simulink model "MX106"  (R2018a)
settings: Solver=VariableStepAuto  StartTime=0.0  StopTime=10.0  RelTol=1e-3
values from neighbouring files (symbols this model uses):
  MX106_amplifier = MX106_supply_voltage/1024    (= 0.014453125)    [MX106_init.m]
  MX106_init_position = 0    [MX106_init.m]
  MX106_Kc = 8e-1    (= 0.8)    [MX106_init.m]
  MX106_Kd = 1/8    (= 0.125)    [MX106_init.m]
  MX106_Ki = 1/1024    (= 0.0009765625)    [MX106_init.m]
  MX106_Kp = 1/4    (= 0.25)    [MX106_init.m]
  MX106_Kv = 9.926e-3    (= 0.009926)    [MX106_init.m]
  MX106_max_speed = 55 * MX106_reduction / 60 * 2 * pi    (= 1468.69456555)    [MX106_init.m]
  MX106_reduction = 255    [MX106_init.m]
  MX106_stall_current = 6.3    [MX106_init.m]
  MX106_stall_torque = 10.0 / MX106_reduction    (= 0.0392156862745)    [MX106_init.m]
  MX106_Te = 1/1000    (= 0.001)    [MX106_init.m]
undefined symbols (not defined in the file or in its folder): MX106_position_gain, MX106_position_offset, MX106_resistor, MX106_speed_gain
libraries: simulink x4, simulink_extras x1, peGeneralControl x1
settings Model: Creator=matt  LastModifiedBy=matt

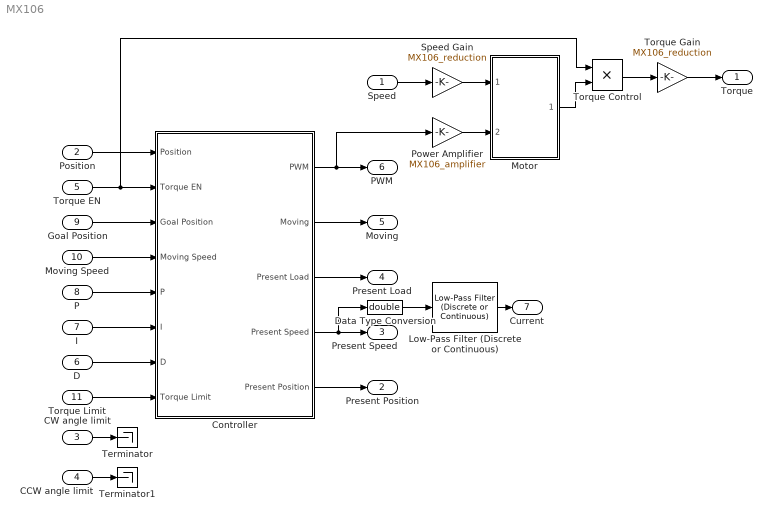
== system MX106 ==
  Speed : Inport
  Position : Inport  Port=2
  CW angle limit : Inport  Port=3  OutDataTypeStr=int16
  CCW angle limit : Inport  Port=4  OutDataTypeStr=int16
  Torque EN : Inport  Port=5  OutDataTypeStr=boolean
  D : Inport  Port=6  OutDataTypeStr=uint8
  I : Inport  Port=7  OutDataTypeStr=uint8
  P : Inport  Port=8  OutDataTypeStr=uint8
  Goal Position : Inport  Port=9
  Moving Speed : Inport  Port=10  OutDataTypeStr=int16
  Torque Limit : Inport  Port=11  OutDataTypeStr=int16
  Controller : Subsystem
  Data Type Conversion : DataTypeConversion  OutDataTypeStr=double
  Low-Pass Filter (Discrete or Continuous) : peGeneralControl/Low-Pass Filter (Discrete or Continuous)  K=9.22996525339537E-07  T=1  B=inf  A=-inf  Ts=-1
  Motor : Subsystem
  Power Amplifier : Gain  Gain=MX106_amplifier  OutDataTypeStr=double
  Speed Gain : Gain  Gain=MX106_reduction
  Terminator : Terminator
  Terminator1 : Terminator
  Torque Control : Product
  Torque Gain : Gain  Gain=MX106_reduction
  Torque : Outport
  Present Position : Outport  Port=2
  Present Speed : Outport  Port=3
  Present Load : Outport  Port=4
  Moving : Outport  Port=5
  PWM : Outport  Port=6
  Current : Outport  Port=7
  wires:
  CW angle limit/1 -> Terminator/1
  CCW angle limit/1 -> Terminator1/1
  Position/1 -> Controller/1(Position)
  Torque EN/1 -> Controller/2(Torque EN), Torque Control/1
  P/1 -> Controller/5(P)
  I/1 -> Controller/6(I)
  D/1 -> Controller/7(D)
  Moving Speed/1 -> Controller/4(Moving Speed)
  Torque Limit/1 -> Controller/8(Torque Limit)
  Controller/2(Moving) -> Moving/1
  Controller/3(Present Load) -> Present Load/1
  Controller/4(Present Speed) -> Data Type Conversion/1, Present Speed/1
  Controller/5(Present Position) -> Present Position/1
  Controller/1(PWM) -> Power Amplifier/1, PWM/1
  Torque Control/1 -> Torque Gain/1
  Speed/1 -> Speed Gain/1
  Speed Gain/1 -> Motor/1(Speed)
  Power Amplifier/1 -> Motor/2(Voltage)
  Motor/1(Torque) -> Torque Control/2
  Goal Position/1 -> Controller/3(Goal Position)
  Torque Gain/1 -> Torque/1
  Low-Pass Filter (Discrete or Continuous)/1 -> Current/1
  Data Type Conversion/1 -> Low-Pass Filter (Discrete or Continuous)/1

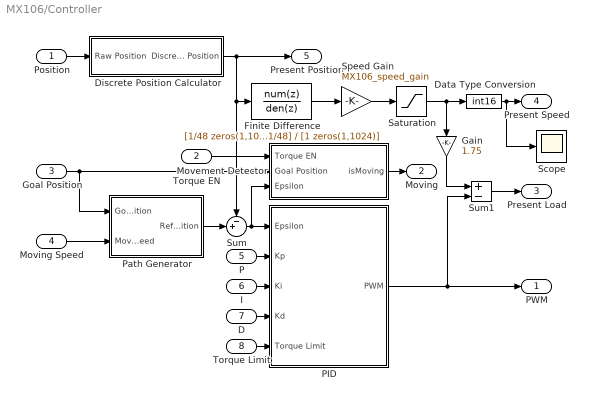
== system MX106/Controller ==
  Position : Inport
  Torque EN : Inport  Port=2
  Goal Position : Inport  Port=3  OutDataTypeStr=int16
  Moving Speed : Inport  Port=4
  P : Inport  Port=5
  I : Inport  Port=6
  D : Inport  Port=7
  Torque Limit : Inport  Port=8
  Data Type Conversion : DataTypeConversion  OutDataTypeStr=int16
  Discrete Position Calculator : Subsystem
  Finite Difference : DiscreteTransferFcn  Numerator=[1/48 zeros(1,1023) -1/48]  Denominator=[1 zeros(1,1024)]  InitialStates=(MX106_init_position + MX106_position_offset) * MX106_position_gain  a0EqualsOne=on
  Gain : Gain  Gain=1.75  OutDataTypeStr=int16
  Movement Detector : Subsystem
  PID : Subsystem
  Path Generator : Subsystem
  Saturation : Saturate  UpperLimit=1024  LowerLimit=-1024  ZeroCross=off
  Scope : Scope
  Speed Gain : Gain  Gain=MX106_speed_gain  OutDataTypeStr=double
  Sum : Sum  Inputs=-+|  AccumDataTypeStr=double  OutMin=-4095  OutMax=4095  OutDataTypeStr=int16  SaturateOnIntegerOverflow=on
  Sum1 : Sum  Inputs=+-
  PWM : Outport
  Moving : Outport  Port=2
  Present Load : Outport  Port=3
  Present Speed : Outport  Port=4
  Present Position : Outport  Port=5
  wires:
  Finite Difference/1 -> Speed Gain/1
  Movement Detector/1(isMoving) -> Moving/1
  Torque EN/1 -> Movement Detector/1(Torque EN)
  Path Generator/1(Ref Position) -> Sum/2
  Moving Speed/1 -> Path Generator/2(Moving Speed)
  Sum/1 -> Movement Detector/3(Epsilon), PID/1(Epsilon)
  Gain/1 -> Sum1/1
  Sum1/1 -> Present Load/1
  P/1 -> PID/2(Kp)
  I/1 -> PID/3(Ki)
  D/1 -> PID/4(Kd)
  Torque Limit/1 -> PID/5(Torque Limit)
  PID/1(PWM) -> Sum1/2, PWM/1
  Data Type Conversion/1 -> Scope/1, Present Speed/1
  Goal Position/1 -> Path Generator/1(Goal Position), Movement Detector/2(Goal Position)
  Discrete Position Calculator/1(Discrete Position) -> Sum/1, Finite Difference/1, Present Position/1
  Position/1 -> Discrete Position Calculator/1(Raw Position)
  Speed Gain/1 -> Saturation/1
  Saturation/1 -> Gain/1, Data Type Conversion/1

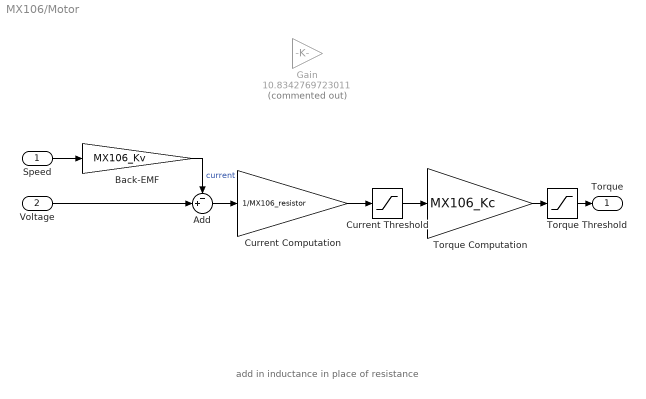
== system MX106/Motor ==
  note: add in inductance in place of resistance
  Speed : Inport
  Voltage : Inport  Port=2
  Add : Sum  Inputs=-+|
  Back-EMF : Gain  Gain=MX106_Kv
  Current Computation : Gain  Gain=1/MX106_resistor
  Current Threshold : Saturate  UpperLimit=MX106_stall_current  LowerLimit=-MX106_stall_current  ZeroCross=off
  Gain : Gain  Commented=on  Gain=10.8342769723011
  Torque Computation : Gain  Gain=MX106_Kc
  Torque Threshold : Saturate  UpperLimit=MX106_stall_torque  LowerLimit=-MX106_stall_torque  ZeroCross=off
  Torque : Outport
  wires:
  Voltage/1 -> Add/2
  Add/1 -> Current Computation/1
  Torque Threshold/1 -> Torque/1
  Current Computation/1 -> Current Threshold/1
  Torque Computation/1 -> Torque Threshold/1
  Current Threshold/1 -> Torque Computation/1
  Back-EMF/1 -> Add/1  "current"
  Speed/1 -> Back-EMF/1

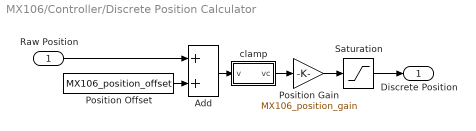
== system MX106/Controller/Discrete Position Calculator ==
  Raw Position : Inport
  Add : Sum
  Position Gain : Gain  Gain=MX106_position_gain  OutMin=0  OutMax=4096  OutDataTypeStr=int16  SampleTime=MX106_Te  SaturateOnIntegerOverflow=on
  Position Offset : Constant  Value=MX106_position_offset
  Saturation : Saturate  UpperLimit=4095  LowerLimit=0  ZeroCross=off
  clamp : Subsystem
  Discrete Position : Outport
  wires:
  Position Gain/1 -> Saturation/1
  Position Offset/1 -> Add/2
  Raw Position/1 -> Add/1
  Saturation/1 -> Discrete Position/1
  Add/1 -> clamp/1(v)
  clamp/1(vc) -> Position Gain/1

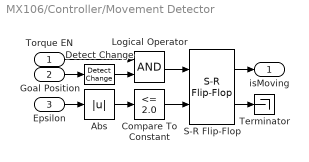
== system MX106/Controller/Movement Detector ==
  Torque EN : Inport
  Goal Position : Inport  Port=2
  Epsilon : Inport  Port=3
  Abs : Abs  ZeroCross=off
  Compare To Constant : simulink/Logic and Bit Operations/Compare To Constant  relop=<=  const=2.0  OutDataTypeStr=boolean  ZeroCross=off
  Detect Change : simulink/Logic and Bit Operations/Detect Change  vinit=0  OutDataTypeStr=boolean
  Logical Operator : Logic  AllPortsSameDT=off  OutDataTypeStr=boolean
  S-R Flip-Flop : simulink_extras/Flip Flops/S-R Flip-Flop  initial_condition=0
  Terminator : Terminator
  isMoving : Outport
  wires:
  Compare To Constant/1 -> S-R Flip-Flop/2
  Abs/1 -> Compare To Constant/1
  Goal Position/1 -> Detect Change/1
  Detect Change/1 -> Logical Operator/2
  S-R Flip-Flop/2 -> Terminator/1
  Logical Operator/1 -> S-R Flip-Flop/1
  Epsilon/1 -> Abs/1
  S-R Flip-Flop/1 -> isMoving/1
  Torque EN/1 -> Logical Operator/1

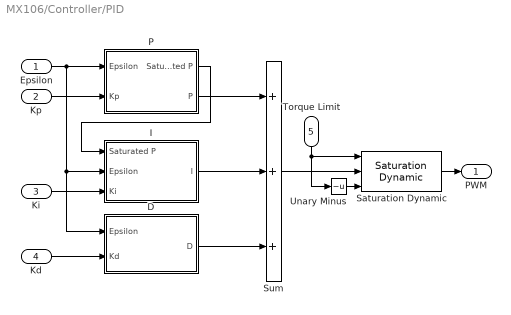
== system MX106/Controller/PID ==
  Epsilon : Inport
  Kp : Inport  Port=2
  Ki : Inport  Port=3
  Kd : Inport  Port=4
  Torque Limit : Inport  Port=5
  D : Subsystem
  I : Subsystem
  P : Subsystem
  Saturation Dynamic : simulink/Discontinuities/Saturation Dynamic  OutMin=[]  OutMax=[]  OutDataTypeStr=Inherit: Same as second input  OutDataType=fixdt(1, 16)  OutScaling=2^-10  DoSatur=off
  Sum : Sum  Inputs=3  OutDataTypeStr=int16  SaturateOnIntegerOverflow=on
  Unary Minus : UnaryMinus
  PWM : Outport
  wires:
  Saturation Dynamic/1 -> PWM/1
  Unary Minus/1 -> Saturation Dynamic/3
  Torque Limit/1 -> Unary Minus/1, Saturation Dynamic/1
  Sum/1 -> Saturation Dynamic/2
  Epsilon/1 -> P/1(Epsilon), D/1(Epsilon), I/2(Epsilon)
  Kp/1 -> P/2(Kp)
  P/2(P) -> Sum/1
  P/1(Saturated P) -> I/1(Saturated P)
  Ki/1 -> I/3(Ki)
  I/1(I) -> Sum/2
  Kd/1 -> D/2(Kd)
  D/1(D) -> Sum/3

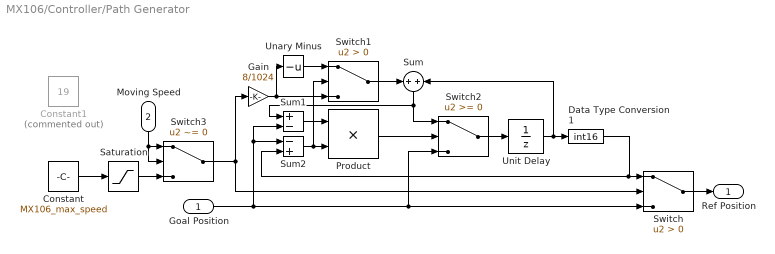
== system MX106/Controller/Path Generator ==
  Goal Position : Inport
  Moving Speed : Inport  Port=2
  Constant : Constant  Value=MX106_max_speed
  Constant1 : Constant  Commented=on  Value=19
  Data Type Conversion1 : DataTypeConversion  OutDataTypeStr=int16
  Gain : Gain  Gain=8/1024  ParamDataTypeStr=double
  Product : Product
  Saturation : Saturate  UpperLimit=1023  LowerLimit=0  ZeroCross=off
  Sum : Sum  Inputs=+|+
  Sum1 : Sum  Inputs=+-
  Sum2 : Sum  Inputs=-+
  Switch : Switch  Criteria=u2 > Threshold  ZeroCross=off
  Switch1 : Switch  Criteria=u2 > Threshold  ZeroCross=off
  Switch2 : Switch  ZeroCross=off
  Switch3 : Switch  Criteria=u2 ~= 0  ZeroCross=off
  Unary Minus : UnaryMinus
  Unit Delay : UnitDelay  InitialCondition=(MX106_init_position + MX106_position_offset) * MX106_position_gain  SampleTime=-1
  Ref Position : Outport
  wires:
  Sum/1 -> Switch2/1, Sum1/1
  Switch/1 -> Ref Position/1
  Switch2/1 -> Unit Delay/1
  Unit Delay/1 -> Sum/2, Data Type Conversion1/1
  Switch1/1 -> Sum/1
  Data Type Conversion1/1 -> Sum2/2, Switch/1
  Sum1/1 -> Product/1
  Sum2/1 -> Switch1/2, Product/2
  Product/1 -> Switch2/2
  Goal Position/1 -> Sum2/1, Sum1/2, Switch2/3, Switch/3
  Unary Minus/1 -> Switch1/1
  Gain/1 -> Switch1/3, Unary Minus/1
  Switch3/1 -> Switch/2, Gain/1
  Moving Speed/1 -> Switch3/2, Switch3/1
  Saturation/1 -> Switch3/3
  Constant/1 -> Saturation/1

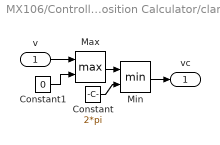
== system MX106/Controller/Discrete Position Calculator/clamp ==
  v : Inport
  Constant : Constant  Value=2*pi
  Constant1 : Constant  Value=0
  Max : MinMax  Function=max  Inputs=2
  Min : MinMax  Inputs=2
  vc : Outport
  wires:
  Constant1/1 -> Max/2
  Min/1 -> vc/1
  v/1 -> Max/1
  Max/1 -> Min/1
  Constant/1 -> Min/2

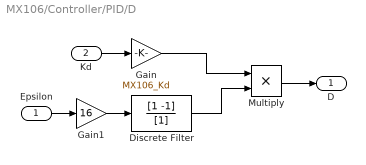
== system MX106/Controller/PID/D ==
  Epsilon : Inport
  Kd : Inport  Port=2
  Discrete Filter : DiscreteFilter  Numerator=[1 -1]  Denominator=[1]
  Gain : Gain  Gain=MX106_Kd  OutDataTypeStr=double
  Gain1 : Gain  Gain=16
  Multiply : Product
  D : Outport
  wires:
  Discrete Filter/1 -> Multiply/2
  Kd/1 -> Gain/1
  Epsilon/1 -> Gain1/1
  Gain/1 -> Multiply/1
  Multiply/1 -> D/1
  Gain1/1 -> Discrete Filter/1

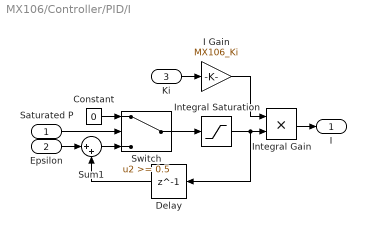
== system MX106/Controller/PID/I ==
  Saturated P : Inport
  Epsilon : Inport  Port=2
  Ki : Inport  Port=3
  Constant : Constant  Value=0
  Delay : Delay  DelayLength=1  SampleTime=MX106_Te
  I Gain : Gain  Gain=MX106_Ki  OutDataTypeStr=double
  Integral Gain : Product
  Integral Saturation : Saturate  UpperLimit=30690  LowerLimit=-30690  ZeroCross=off
  Sum1 : Sum  Inputs=|++
  Switch : Switch  Threshold=0.5  ZeroCross=off
  I : Outport
  wires:
  Saturated P/1 -> Switch/2
  I Gain/1 -> Integral Gain/1
  Ki/1 -> I Gain/1
  Constant/1 -> Switch/1
  Switch/1 -> Integral Saturation/1
  Epsilon/1 -> Sum1/1
  Integral Gain/1 -> I/1
  Delay/1 -> Sum1/2
  Sum1/1 -> Switch/3
  Integral Saturation/1 -> Delay/1, Integral Gain/2

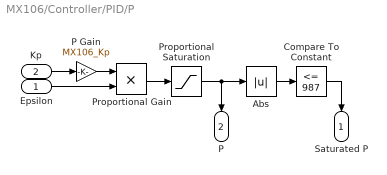
== system MX106/Controller/PID/P ==
  Epsilon : Inport
  Kp : Inport  Port=2
  Abs : Abs  ZeroCross=off
  Compare To Constant : simulink/Logic and Bit Operations/Compare To Constant  relop=<=  const=987  OutDataTypeStr=boolean  ZeroCross=off
  P Gain : Gain  Gain=MX106_Kp  OutDataTypeStr=double
  Proportional Gain : Product
  Proportional Saturation : Saturate  UpperLimit=987  LowerLimit=-987  ZeroCross=off
  Saturated P : Outport
  P : Outport  Port=2
  wires:
  P Gain/1 -> Proportional Gain/1
  Abs/1 -> Compare To Constant/1
  Epsilon/1 -> Proportional Gain/2
  Proportional Saturation/1 -> Abs/1, P/1
  Compare To Constant/1 -> Saturated P/1
  Proportional Gain/1 -> Proportional Saturation/1
  Kp/1 -> P Gain/1
